simulink model "Exercitiul_5"  (R2021b)
settings: Solver=VariableStepAuto  StartTime=0.0  StopTime=10.0  RelTol=1e-3
libraries: simulink x1
settings Model: Creator=Petrisor  LastModifiedBy=Petrisor

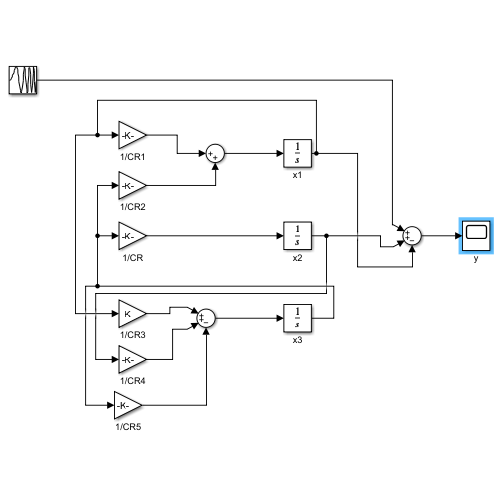
[thumbnail: Simulink's stored preview of the top-level diagram]
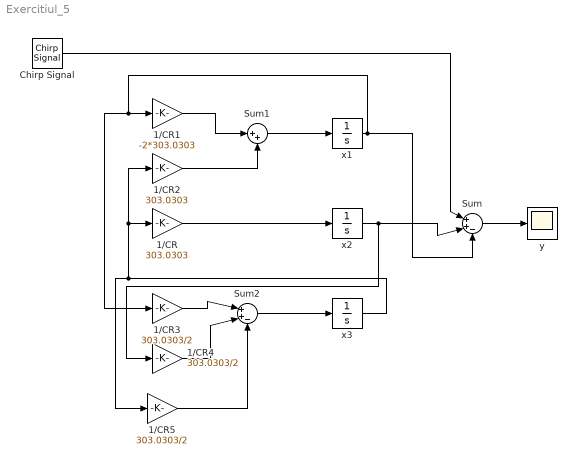
== system Exercitiul_5 ==
  1/CR : Gain  Gain=303.0303
  1/CR1 : Gain  Gain=-2*303.0303
  1/CR2 : Gain  Gain=303.0303
  1/CR3 : Gain  Gain=303.0303/2
  1/CR4 : Gain  Gain=303.0303/2
  1/CR5 : Gain  Gain=303.0303/2
  Chirp Signal : simulink/Sources/Chirp Signal  f1=0.1  T=300  f2=10
  Sum : Sum  Inputs=|++-
  Sum1 : Sum  Inputs=|++
  Sum2 : Sum  Inputs=|++-
  x1 : Integrator
  x2 : Integrator
  x3 : Integrator
  y : Scope
  wires:
  Sum/1 -> y/1
  x1/1 -> 1/CR3/1, 1/CR1/1, Sum/3
  x2/1 -> 1/CR4/1, Sum/2
  Chirp Signal/1 -> Sum/1
  x3/1 -> 1/CR5/1, 1/CR2/1, 1/CR/1
  1/CR/1 -> x2/1
  1/CR1/1 -> Sum1/1
  1/CR2/1 -> Sum1/2
  Sum1/1 -> x1/1
  Sum2/1 -> x3/1
  1/CR3/1 -> Sum2/1
  1/CR4/1 -> Sum2/2
  1/CR5/1 -> Sum2/3
